simulink subsystem "torquelimit"  (R2022b)
settings: Solver=VariableStepAuto  StartTime=0.0  StopTime=10.0  RelTol=1e-3
libraries: simulink x2
settings Model: Creator=serga  LastModifiedBy=serga

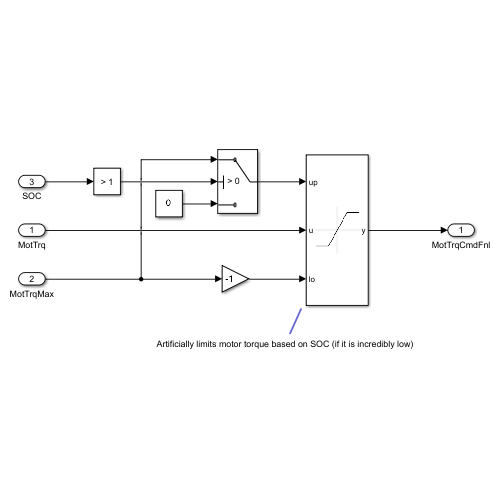
[thumbnail: Simulink's stored preview of the top-level diagram]
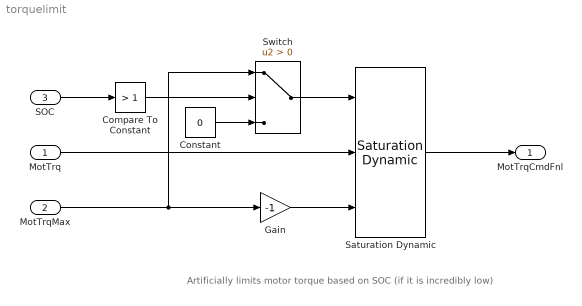
== system torquelimit ==
  note: Artificially limits motor torque based on SOC (if it is incredibly low)
  MotTrq : Inport
  MotTrqMax : Inport  Port=2
  SOC : Inport  Port=3
  Compare To Constant : simulink/Logic and Bit Operations/Compare To Constant  relop=>  const=1  OutDataTypeStr=boolean
  Constant : Constant  Value=0
  Gain : Gain  Gain=-1
  Saturation Dynamic : simulink/Discontinuities/Saturation Dynamic  OutMin=[]  OutMax=[]  OutDataTypeStr=Inherit: Same as second input  OutDataType=fixdt(1, 16)  OutScaling=2^-10  DoSatur=off
  Switch : Switch  Criteria=u2 > Threshold  SaturateOnIntegerOverflow=off  InputSameDT=off
  MotTrqCmdFnl : Outport
  wires:
  Compare To Constant/1 -> Switch/2
  SOC/1 -> Compare To Constant/1
  Switch/1 -> Saturation Dynamic/1
  Saturation Dynamic/1 -> MotTrqCmdFnl/1
  Gain/1 -> Saturation Dynamic/3
  MotTrq/1 -> Saturation Dynamic/2
  MotTrqMax/1 -> Gain/1, Switch/1
  Constant/1 -> Switch/3
